simulink model "c12_AdapMultipleDelayConsensus"  (R2022b)
settings: Solver=VariableStepAuto  StartTime=0.0  StopTime=t_end  RelTol=1e-6
values from neighbouring files (symbols this model uses):
  a0 = 1/5    (= 0.2)    [c12_delayAdaptive.m]
  L1 = Hbar1'*W*Hbar1    [c12_MultipleDelaysLMI.m]
  L2 = Hbar2'*W*Hbar2    [c12_MultipleDelaysLMI.m]
  L3 = Hbar3'*W*Hbar3    [c12_MultipleDelaysLMI.m]
  x0 = 5    [c12_delayAdaptive.m]    (also in c14_bipartite_MWconsensus_animation.m = [x0;r/norm(r)]; c15_closed_model.m = 5*rand(15,1); c15_open_model.m = 5*rand(15,1))
undefined symbols (not defined in the file or in its folder): tau1, tau2, tau3
settings Model: Creator=trinh  LastModifiedBy=trinh
settings SolverCC: ZeroCrossAlgorithm=Adaptive

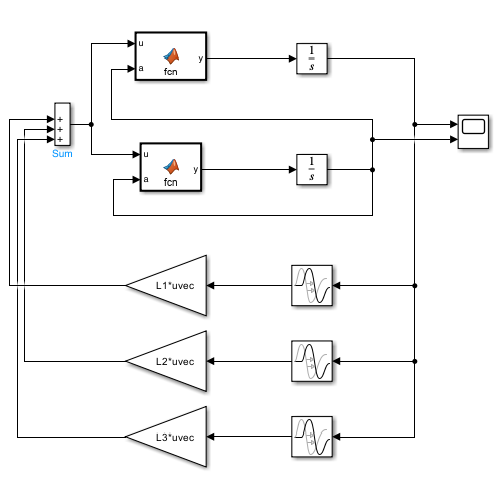
[thumbnail: Simulink's stored preview of the top-level diagram]
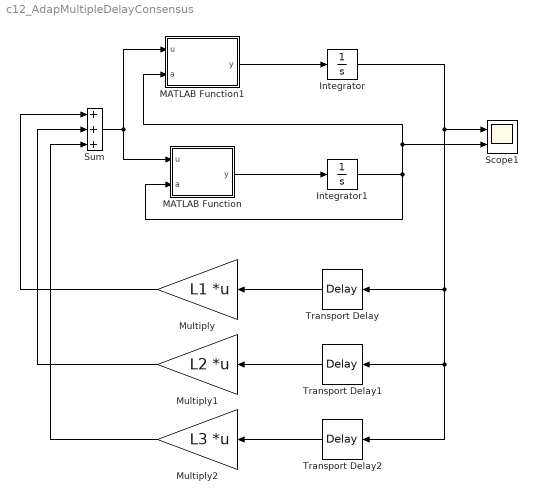
== system c12_AdapMultipleDelayConsensus ==
  Integrator : Integrator  InitialCondition=x0
  Integrator1 : Integrator  InitialCondition=a0
  MATLAB Function : MATLAB Function  TreatAsAtomicUnit=on
  MATLAB Function1 : MATLAB Function  TreatAsAtomicUnit=on
  Multiply : Gain  Gain=L1  Multiplication=Matrix(K*u) (u vector)
  Multiply1 : Gain  Gain=L2  Multiplication=Matrix(K*u) (u vector)
  Multiply2 : Gain  Gain=L3  Multiplication=Matrix(K*u) (u vector)
  Scope1 : Scope  NumInputPorts=2
  Sum : Sum  Inputs=|+++
  Transport Delay : TransportDelay  DelayTime=tau1
  Transport Delay1 : TransportDelay  DelayTime=tau2
  Transport Delay2 : TransportDelay  DelayTime=tau3
  wires:
  Integrator/1 -> Scope1/1, Transport Delay2/1, Transport Delay1/1, Transport Delay/1
  MATLAB Function1/1(y) -> Integrator/1
  Transport Delay/1 -> Multiply/1
  Multiply/1 -> Sum/1
  MATLAB Function/1(y) -> Integrator1/1
  Integrator1/1 -> MATLAB Function/2(a), Scope1/2, MATLAB Function1/2(a)
  Multiply1/1 -> Sum/2
  Transport Delay1/1 -> Multiply1/1
  Transport Delay2/1 -> Multiply2/1
  Multiply2/1 -> Sum/3
  Sum/1 -> MATLAB Function/1(u), MATLAB Function1/1(u)

== matlab function c12_AdapMultipleDelayConsensus/MATLAB Function1 ==
  data: u input; y output; a input
function y = fcn(u,a)
    y = -inv(kron(diag(a),eye(3)))*u;
end

== matlab function c12_AdapMultipleDelayConsensus/MATLAB Function ==
  data: u input; y output; a input
function y= fcn(u,a)
gamma = ones(9,1)*0.1;
y1 = gamma(1)*norm(u(1:3),2)/a(1);
y2 = gamma(2)*norm(u(4:6),2)/a(2);
y3 = gamma(3)*norm(u(7:9),2)/a(3);
y4 = gamma(4)*norm(u(10:12),2)/a(4);
y5 = gamma(5)*norm(u(13:15),2)/a(5);
y6 = gamma(6)*norm(u(16:18),2)/a(6);
y7 = gamma(7)*norm(u(19:21),2)/a(7);
y8 = gamma(8)*norm(u(22:24),2)/a(8);
y9 = gamma(9)*norm(u(25:27),2)/a(9);
y = [y1;y2;y3;y4;y5;y6;y7;y8;y9];
end
